simulink model "BatterySimulationCCCV"  (R2018b)
settings: Solver=FixedStepAuto  StartTime=0.0  StopTime=10.0  FixedStep=0.01  MaxStep=0.01  MinStep=0.01  RelTol=1e-3
settings Model: Creator=GRosp  LastModifiedBy=GRosp

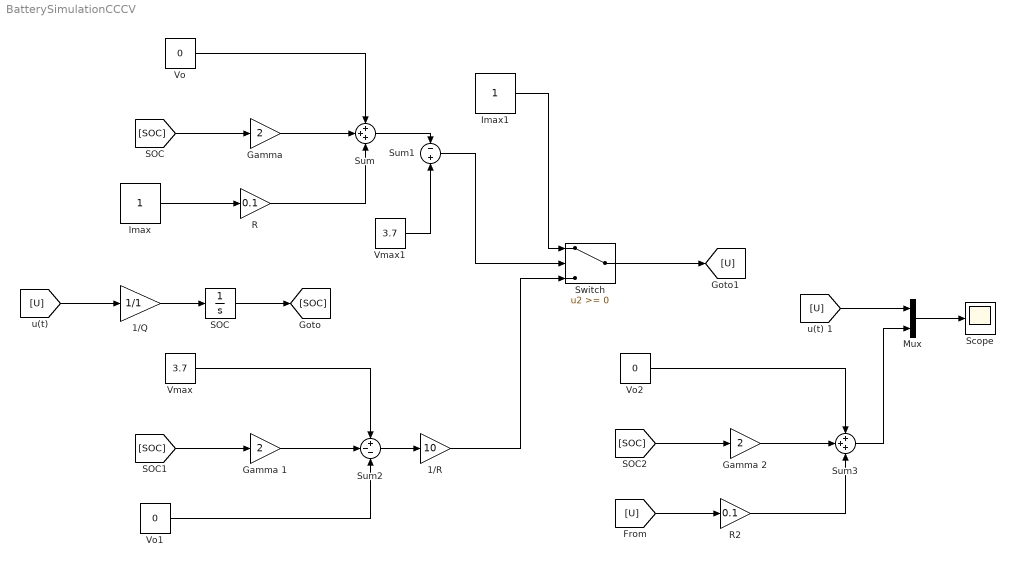
== system BatterySimulationCCCV ==
  1/Q : Gain  Gain=1/1
  "1/R " : Gain  Gain=10
  "Gamma " : Gain  Gain=2
  Gamma 1 : Gain  Gain=2
  Gamma 2 : Gain  Gain=2
  Imax : Constant
  Imax1 : Constant
  Mux : Mux  Inputs=2
  R : Gain  Gain=0.1
  R2 : Gain  Gain=0.1
  "SOC " : Integrator
  Scope : Scope
  Sum : Sum  Inputs=+++
  Sum1 : Sum  Inputs=-+
  Sum2 : Sum  Inputs=+--
  Sum3 : Sum  Inputs=+++
  Switch : Switch
  Vmax : Constant  Value=3.7
  "Vmax1 " : Constant  Value=3.7
  Vo : Constant  Value=0
  Vo1 : Constant  Value=0
  Vo2 : Constant  Value=0
  wires:
  Vo/1 -> Sum/1
  1/Q/1 -> "SOC "/1
  [U] -> 1/Q/1
  "SOC "/1 -> [SOC]
  Imax/1 -> R/1
  R/1 -> Sum/3
  Imax1/1 -> Switch/1
  [SOC] -> "Gamma "/1
  "Gamma "/1 -> Sum/2
  Sum/1 -> Sum1/1
  "Vmax1 "/1 -> Sum1/2
  Sum1/1 -> Switch/2
  Switch/1 -> [U]
  [SOC] -> Gamma 1/1
  Gamma 1/1 -> Sum2/2
  Vmax/1 -> Sum2/1
  [SOC] -> Gamma 2/1
  R2/1 -> Sum3/3
  Gamma 2/1 -> Sum3/2
  Vo2/1 -> Sum3/1
  Sum2/1 -> "1/R "/1
  "1/R "/1 -> Switch/3
  Vo1/1 -> Sum2/3
  [U] -> R2/1
  Sum3/1 -> Mux/2
  [U] -> Mux/1
  Mux/1 -> Scope/1
